simulink library "satEulerDyn_sl"  (R2023b)
settings: Solver=VariableStepAuto  StartTime=0.0  StopTime=10.0  RelTol=1e-3
undefined symbols (not defined in the file): satInertiaTensor
settings Model: Creator=gilbu  LastModifiedBy=gilbu

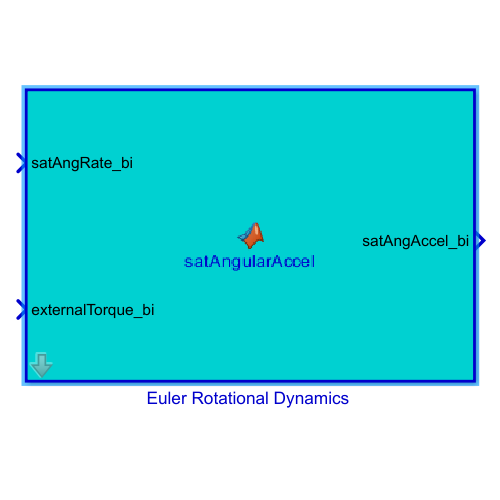
[thumbnail: Simulink's stored preview of the top-level diagram]
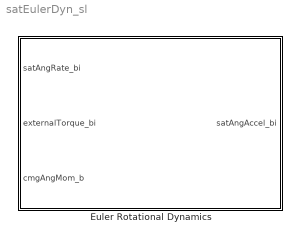
== system satEulerDyn_sl ==
  "Euler Rotational Dynamics " : MATLAB Function  TreatAsAtomicUnit=on  mask{satInertiaTensor=satInertiaTensor}
      mask prompts: satInertiaTensor "Satellite Inertia Tensor <3,3> [kg*m^2]"

== matlab function satEulerDyn_sl/Euler Rotational Dynamics  ==
  data: satAngRate_bi input size=3; externalTorque_bi input size=3; cmgAngMom_b input size=3; satAngAccel_bi output size=3; satInertiaTensor parameter size=3,3
%satAngularAccel   Rigid Body Dynamics for Satellite under angular accel.
function satAngAccel_bi = satAngularAccel( ...
    satAngRate_bi,externalTorque_bi,cmgAngMom_b, ...% Inputs
    satInertiaTensor ... % Parameters
    )

% ------------------------------------------------------------------------------
% Calculate Angular Acceleration

% if norm(cmgAngMom_b) >= 4760*4
%     [M,i] = max(cmgAngMom_b);
%     deSatTorque = [0;0;0];
%     deSatTorque(i) = -M/0.1;
%else
    deSatTorque = [0;0;0];
%end
satAngAccel_bi = satInertiaTensor\-cross(satAngRate_bi,satInertiaTensor*satAngRate_bi+cmgAngMom_b)+satInertiaTensor\externalTorque_bi + satInertiaTensor\deSatTorque;


end
